simulink library "Lib_PF_ActiveConvEffDC2DC_TMATS"  (R2020b)
settings: Solver=ode45  StartTime=0.0  StopTime=10.0  RelTol=1e-3  EnableMultiTasking=on
Description:
  | Thomas Modules
settings Model: Creator=jwchapm2  LastModifiedBy=mebell
settings DataIOCC: LimitDataPoints=on  SaveFormat=Array  ReturnWorkspaceOutputs=off
settings OptimizationCC: ExpressionDepthLimit=2147483647  LifeSpan=inf
settings DebuggingCC: UnderspecifiedInitializationDetection=Classic  MergeDetectMultiDrivingBlocksExec=none  SolverPrmCheckMsg=warning  StateNameClashWarn=warning  SFUnexpectedBacktrackingDiag=warning  SFNoUnconditionalDefaultTransitionDiag=warning  SFExecutionAtInitializationDiag=none  ArithmeticOperatorsInVariantConditions=warning
settings HardwareCC: ProdBitPerPointer=32  ProdBitPerSizeT=32  ProdBitPerPtrDiffT=32  ProdLargestAtomicFloat=None  ProdIntDivRoundTo=Undefined  ProdEndianess=Unspecified  ProdWordSize=32  ProdHWDeviceType=32-bit Generic
settings ModelReferenceCC: PropagateSignalLabelsOutOfModel=off
settings SFSimCC: SimUseLocalCustomCode=off  CustomCodeUndefinedFunction=UseInterfaceOnly
settings RTWCC: RTWUseLocalCustomCode=off
settings CodeAppCC: StateflowObjectComments=on
settings GRTTargetCC: TargetLangStandard=C89/C90 (ANSI)
settings ConfigComp: CovMetricSettings=dw  CovSaveCumulativeToWorkspaceVar=on  CovSaveSingleToWorkspaceVar=on  CovExternalEMLEnable=off

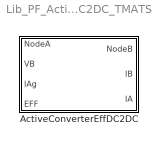
== system Lib_PF_ActiveConvEffDC2DC_TMATS ==
  ActiveConverterEffDC2DC : Subsystem  mask{BlkNm_M=double(gcb)}
      mask prompts: BlkNm_M "Block name as double for simulink output"
      mask Display:
      | fprintf('DC : DC')
      | port_label('input',1,'VA')
      | port_label('input',2,'VB')
      | port_label('input',3,'IAg')
      | port_label('input',4,'Eff')
      | port_label('output',1,'VB')
      | port_label('output',2,'IB')
      | port_label('output',3,'IA')

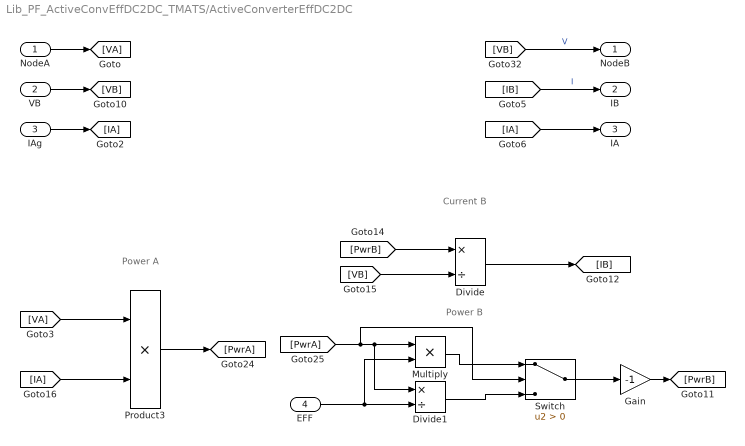
== system Lib_PF_ActiveConvEffDC2DC_TMATS/ActiveConverterEffDC2DC ==
  note: Power A
  note: Current B
  note: Power B
  NodeA : Inport
  VB : Inport  Port=2
  IAg : Inport  Port=3
  EFF : Inport  Port=4
  Divide : Product  Inputs=*/
  Divide1 : Product  Inputs=*/
  Gain : Gain  Gain=-1
  Multiply : Product
  Product3 : Product
  Switch : Switch  Criteria=u2 > Threshold
  NodeB : Outport  VectorParamsAs1DForOutWhenUnconnected=off
  IB : Outport  Port=2  VectorParamsAs1DForOutWhenUnconnected=off
  IA : Outport  Port=3  VectorParamsAs1DForOutWhenUnconnected=off
  wires:
  [VA] -> Product3/1
  Product3/1 -> [PwrA]
  [VB] -> NodeB/1  "V"
  NodeA/1 -> [VA]
  [IA] -> Product3/2
  Gain/1 -> [PwrB]
  [PwrB] -> Divide/1
  Switch/1 -> Gain/1
  [PwrA] -> Switch/2, Divide1/1, Multiply/1
  Divide/1 -> [IB]
  [VB] -> Divide/2
  IAg/1 -> [IA]
  [IB] -> IB/1  "I"
  EFF/1 -> Multiply/2, Divide1/2
  VB/1 -> [VB]
  [IA] -> IA/1
  Divide1/1 -> Switch/3
  Multiply/1 -> Switch/1
